simulink model "No3_RWSerialData"  (R2022a)
settings: Solver=FixedStepAuto  StartTime=0.0  StopTime=inf  MaxStep=0.005  RelTol=1e-3  EnableMultiTasking=on
libraries: px4uORBlib x2, px4lib x2, etargetslib x1
settings Model: ExtModeTrigDuration=10  Creator=liuwhale  LastModifiedBy=liuwhale
settings SolverCC: PositivePriorityOrder=on
settings OptimizationCC: EnhancedBackFolding=on  PassReuseOutputArgsAs=Individual arguments  ZeroExternalMemoryAtStartup=off  ZeroInternalMemoryAtStartup=off  MaxStackSize=64  OptimizeBlockOrder=speed  DifferentSizesBufferReuse=on  OptimizationCustomize=off  EfficientTunableParamExpr=on
settings DebuggingCC: ParameterTunabilityLossMsg=error
settings HardwareCC: ProdBitPerPointer=32  ProdBitPerSizeT=32  ProdBitPerPtrDiffT=32  ProdLargestAtomicInteger=Long  ProdLargestAtomicFloat=Double  ProdWordSize=32  ProdLongLongMode=on  ProdHWDeviceType=ARM Compatible->ARM Cortex
settings SFSimCC: MATLABDynamicMemAlloc=off  SimTargetLang=C++
settings RTWCC: SystemTargetFile=ert.tlc  HardwareBoard=PX4 Pixhawk 1  TLCOptions="-aInlineSetEventsForThisBaseRateFcn=TLC_FALSE -aSuppressMultiTaskScheduler=TLC_FALSE  -aRateBasedStepFcn=0"  TemplateMakefile=ert_default_tmf  Toolchain=GNU Tools for PX4 Autopilots  TargetLang=C++
settings CodeAppCC: ForceParamTrailComments=on  IgnoreCustomStorageClasses=off  OperatorAnnotations=on  SimulinkDataObjDesc=on  SFDataObjDesc=on  InsertBlockDesc=on
settings ERTTargetCC: ExtModeStaticAllocSize=1024

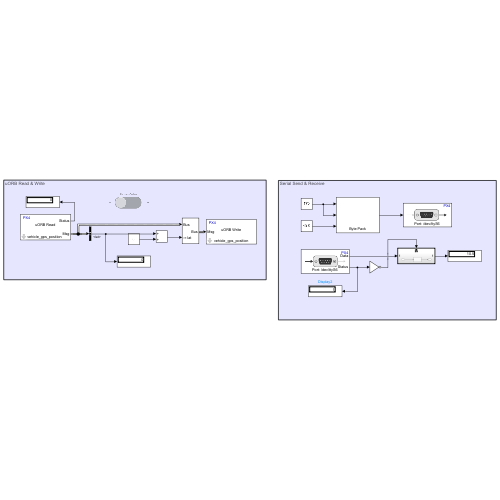
[thumbnail: Simulink's stored preview of the top-level diagram]
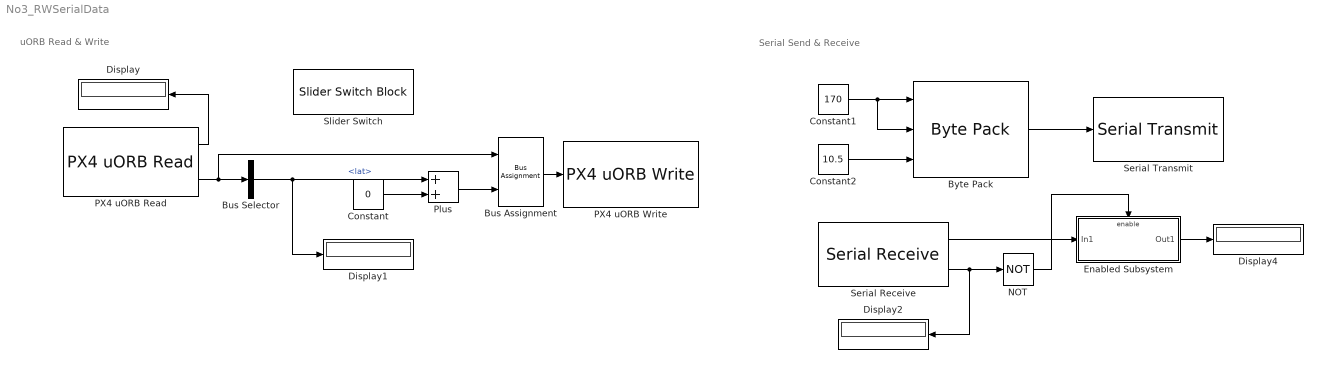
== system No3_RWSerialData ==
  note: Serial Send & Receive
  note: uORB Read & Write
  Bus Assignment : BusAssignment  AssignedSignals=lat
  Bus Selector : BusSelector  OutputSignals=lat
  Byte Pack : etargetslib/Byte Pack  datatypes={'uint8','uint8','double'}  byteAlign=1
  Constant : Constant  Value=0
  Constant1 : Constant  Value=170  OutDataTypeStr=uint8
  Constant2 : Constant  Value=10.5  OutDataTypeStr=double
  Display{,1..2,4} (4 alike) : Display
  Enabled Subsystem : Subsystem  TreatAsAtomicUnit=on
  NOT : Logic  Operator=NOT  IconShape=distinctive  AllPortsSameDT=off  OutDataTypeStr=boolean
  PX4 uORB Read : px4uORBlib/PX4 uORB Read  uORBTopic=vehicle_gps_position  selectInstance=vehicle_gps_position  SampleTime=-1  BlockingMode=off  BlockTimeout=1e-3
      settings: SourceProductBaseCode=PX4AUTOPILOTS
  PX4 uORB Write : px4uORBlib/PX4 uORB Write  uORBTopic=vehicle_gps_position  selectInstance=vehicle_gps_position  MessageQueueLen=1
      settings: SourceProductBaseCode=PX4AUTOPILOTS
  Plus : Sum  OutDataTypeStr=int32
  Serial Receive : px4lib/Serial Receive  SCIModule=/dev/ttyS6  DataType=uint8  DataLength=20  OutputStatus=on  SampleTime=0.1  BlockingMode=off  PartialData=off  Timeout=5
      settings: SourceProductBaseCode=PX4AUTOPILOTS
  Serial Transmit : px4lib/Serial Transmit  SCIModule=/dev/ttyS6
      settings: SourceProductBaseCode=PX4AUTOPILOTS
  Slider Switch : SliderSwitchBlock
      settings: Values={{'Off', 'On'}, [0 1]}
  wires:
  PX4 uORB Read/1 -> Display/1
  PX4 uORB Read/2 -> Bus Assignment/1, Bus Selector/1
  Bus Selector/1 -> Display1/1, Plus/1  "<lat>"
  Bus Assignment/1 -> PX4 uORB Write/1
  Plus/1 -> Bus Assignment/2
  Constant/1 -> Plus/2
  Byte Pack/1 -> Serial Transmit/1
  Constant1/1 -> Byte Pack/1, Byte Pack/2
  Constant2/1 -> Byte Pack/3
  Serial Receive/2 -> NOT/1, Display2/1
  Serial Receive/1 -> Enabled Subsystem/1(In1)
  NOT/1 -> Enabled Subsystem/Enable
  Enabled Subsystem/1(Out1) -> Display4/1

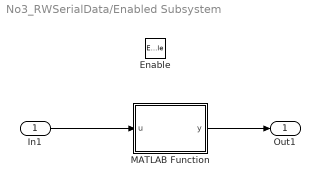
== system No3_RWSerialData/Enabled Subsystem ==
  In1 : Inport
  Enable : EnablePort
  MATLAB Function : MATLAB Function  TreatAsAtomicUnit=on
  Out1 : Outport
  wires:
  In1/1 -> MATLAB Function/1(u)
  MATLAB Function/1(y) -> Out1/1

== matlab function No3_RWSerialData/Enabled Subsystem/MATLAB Function ==
  data: u input; y output
function y = fcn(u)
  y = zeros(1,1);
    for i = 1:20
        if i < 12
            if u(i) == 170 && u(i + 1) == 170
                y(1) = typecast( uint8([u(i + 2),u(i + 3),u(i + 4),u(i + 5), u(i + 6),u(i + 7),u(i + 8),u(i + 9)]),'double');
            end
        end
    end
